simulink model "Test_model_Froce"  (R2024a)
settings: Solver=VariableStepAuto  StartTime=0.0  StopTime=inf  RelTol=1e-3
undefined symbols (not defined in the file or in its folder): X, Y, Z
libraries: sm_lib x62, nesl_utility x21, robotcorelib x4, simulink x1
(part 3 of 3)

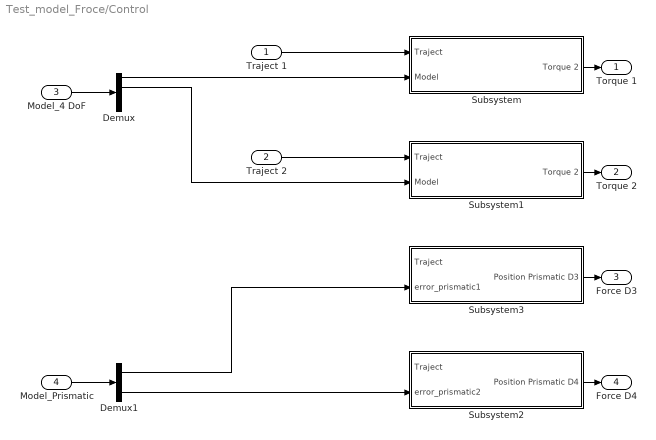
== system Test_model_Froce/Control ==
  Traject 1 : Inport
  Traject 2 : Inport  Port=2
  Model_4 DoF : Inport  Port=3
  Model_Prismatic : Inport  Port=4
  Demux : Demux
  Demux1 : Demux  Outputs=2
  Subsystem : Subsystem
  Subsystem1 : Subsystem
  Subsystem2 : Subsystem
  Subsystem3 : Subsystem
  Torque 1 : Outport
  Torque 2 : Outport  Port=2
  Force D3 : Outport  Port=3
  Force D4 : Outport  Port=4
  wires:
  Subsystem1/1(Torque 2) -> Torque 2/1
  Subsystem/1(Torque 2) -> Torque 1/1
  Subsystem3/1(Position Prismatic D3) -> Force D3/1
  Subsystem2/1(Position Prismatic D4) -> Force D4/1
  Model_4 DoF/1 -> Demux/1
  Demux/1 -> Subsystem/2(Model)
  Demux/2 -> Subsystem1/2(Model)
  Traject 1/1 -> Subsystem/1(Traject)
  Traject 2/1 -> Subsystem1/1(Traject)
  Model_Prismatic/1 -> Demux1/1
  Demux1/1 -> Subsystem3/2(error_prismatic1)
  Demux1/2 -> Subsystem2/2(error_prismatic2)

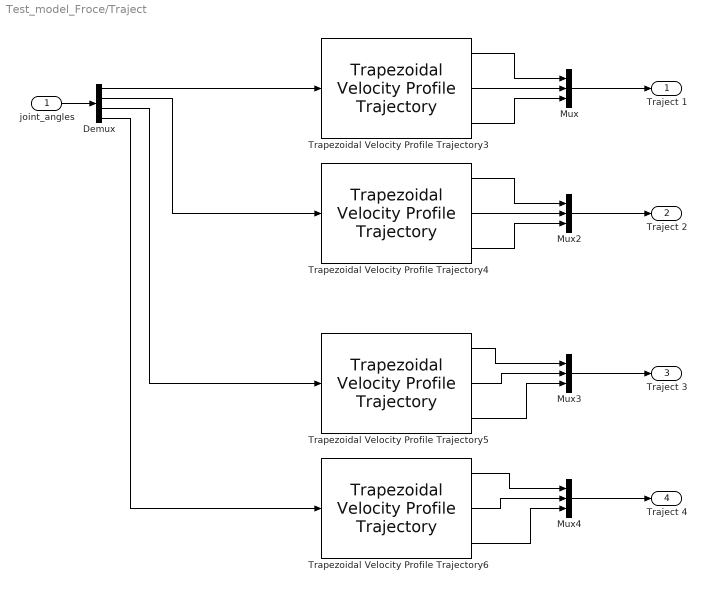
== system Test_model_Froce/Traject ==
  joint_angles : Inport
  Demux : Demux
  Mux{,2..4} (4 alike) : Mux  Inputs=3
  Trapezoidal Velocity Profile Trajectory3 : robotcorelib/Trapezoidal Velocity Profile Trajectory  WaypointSource=Internal  Waypoints=[ 0, 0, 0]  NumParams=0  Parameter1=Peak Velocity  Parameter2=End Time  ParameterSource=Internal  PeakVelocity=[ 2; 2 ]  Acceleration=[ 1; 2 ]  EndTime=[ 1; 1 ]  AccelTime=[ 1; 2 ]  SimulateUsing=Interpreted execution
  Trapezoidal Velocity Profile Trajectory4 : robotcorelib/Trapezoidal Velocity Profile Trajectory  WaypointSource=Internal  Waypoints=[ 0, 0, 0]  NumParams=0  Parameter1=Peak Velocity  Parameter2=End Time  ParameterSource=Internal  PeakVelocity=[ 2; 2 ]  Acceleration=[ 1; 2 ]  EndTime=[ 1; 1 ]  AccelTime=[ 1; 2 ]  SimulateUsing=Interpreted execution
  Trapezoidal Velocity Profile Trajectory5 : robotcorelib/Trapezoidal Velocity Profile Trajectory  WaypointSource=Internal  Waypoints=[ 0, 1, 5]  NumParams=0  Parameter1=Peak Velocity  Parameter2=End Time  ParameterSource=Internal  PeakVelocity=[ 2; 2 ]  Acceleration=[ 1; 2 ]  EndTime=[ 1; 1 ]  AccelTime=[ 1; 2 ]  SimulateUsing=Interpreted execution
  Trapezoidal Velocity Profile Trajectory6 : robotcorelib/Trapezoidal Velocity Profile Trajectory  WaypointSource=Internal  Waypoints=[ 0, 1, 3]  NumParams=0  Parameter1=Peak Velocity  Parameter2=End Time  ParameterSource=Internal  PeakVelocity=[ 2; 2 ]  Acceleration=[ 1; 2 ]  EndTime=[ 1; 1 ]  AccelTime=[ 1; 2 ]  SimulateUsing=Interpreted execution
  Traject 1 : Outport
  Traject 2 : Outport  Port=2
  Traject 3 : Outport  Port=3
  Traject 4 : Outport  Port=4
  wires:
  Trapezoidal Velocity Profile Trajectory5/2 -> Mux3/2
  Trapezoidal Velocity Profile Trajectory3/2 -> Mux/2
  Trapezoidal Velocity Profile Trajectory6/1 -> Mux4/1
  Trapezoidal Velocity Profile Trajectory6/2 -> Mux4/2
  Trapezoidal Velocity Profile Trajectory3/3 -> Mux/3
  Trapezoidal Velocity Profile Trajectory6/3 -> Mux4/3
  Trapezoidal Velocity Profile Trajectory5/3 -> Mux3/3
  Trapezoidal Velocity Profile Trajectory3/1 -> Mux/1
  Trapezoidal Velocity Profile Trajectory4/3 -> Mux2/3
  Trapezoidal Velocity Profile Trajectory4/1 -> Mux2/1
  Trapezoidal Velocity Profile Trajectory4/2 -> Mux2/2
  Trapezoidal Velocity Profile Trajectory5/1 -> Mux3/1
  Mux/1 -> Traject 1/1
  joint_angles/1 -> Demux/1
  Demux/1 -> Trapezoidal Velocity Profile Trajectory3/1
  Demux/2 -> Trapezoidal Velocity Profile Trajectory4/1
  Demux/3 -> Trapezoidal Velocity Profile Trajectory5/1
  Demux/4 -> Trapezoidal Velocity Profile Trajectory6/1
  Mux2/1 -> Traject 2/1
  Mux3/1 -> Traject 3/1
  Mux4/1 -> Traject 4/1

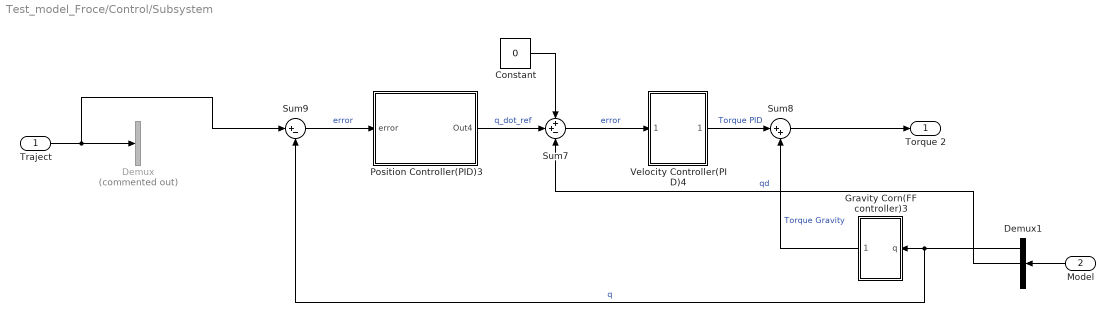
== system Test_model_Froce/Control/Subsystem ==
  Traject : Inport
  Model : Inport  Port=2
  Constant : Constant  Value=0
  Demux : Demux  Commented=on  Outputs=3
  Demux1 : Demux  Outputs=3
  Gravity Corn(FF controller)3 : Subsystem
  Position Controller(PID)3 : Subsystem
  Sum7 : Sum  Inputs=++-
  Sum8 : Sum  Inputs=|++
  Sum9 : Sum  Inputs=|+-
  Velocity Controller(PID)4 : Subsystem
  Torque 2 : Outport
  wires:
  Position Controller(PID)3/1(Out4) -> Sum7/2  "q_dot_ref"
  Gravity Corn(FF controller)3/1(Out1) -> Sum8/2  "Torque Gravity"
  Traject/1 -> Sum9/1, Demux/1
  Velocity Controller(PID)4/1(Out4) -> Sum8/1  "Torque PID"
  Sum7/1 -> Velocity Controller(PID)4/1(error)  "error"
  Sum9/1 -> Position Controller(PID)3/1(error)  "error"
  Sum8/1 -> Torque 2/1
  Model/1 -> Demux1/1
  Demux1/1 -> Sum9/2, Gravity Corn(FF controller)3/1(q)  "q"
  Demux1/2 -> Sum7/3  "qd"
  Constant/1 -> Sum7/1

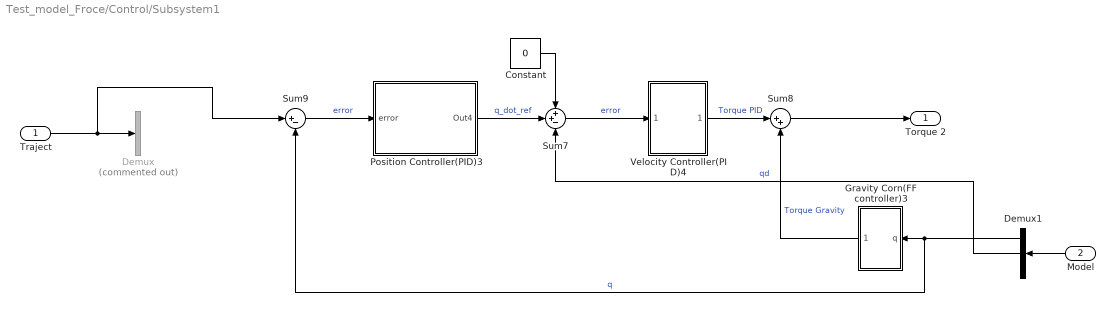
== system Test_model_Froce/Control/Subsystem1 ==
  Traject : Inport
  Model : Inport  Port=2
  Constant : Constant  Value=0
  Demux : Demux  Commented=on  Outputs=3
  Demux1 : Demux  Outputs=3
  Gravity Corn(FF controller)3 : Subsystem
  Position Controller(PID)3 : Subsystem
  Sum7 : Sum  Inputs=++-
  Sum8 : Sum  Inputs=|++
  Sum9 : Sum  Inputs=|+-
  Velocity Controller(PID)4 : Subsystem
  Torque 2 : Outport
  wires:
  Position Controller(PID)3/1(Out4) -> Sum7/2  "q_dot_ref"
  Gravity Corn(FF controller)3/1(Out1) -> Sum8/2  "Torque Gravity"
  Traject/1 -> Sum9/1, Demux/1
  Velocity Controller(PID)4/1(Out4) -> Sum8/1  "Torque PID"
  Sum7/1 -> Velocity Controller(PID)4/1(error)  "error"
  Sum9/1 -> Position Controller(PID)3/1(error)  "error"
  Sum8/1 -> Torque 2/1
  Model/1 -> Demux1/1
  Demux1/1 -> Sum9/2, Gravity Corn(FF controller)3/1(q)  "q"
  Demux1/2 -> Sum7/3  "qd"
  Constant/1 -> Sum7/1

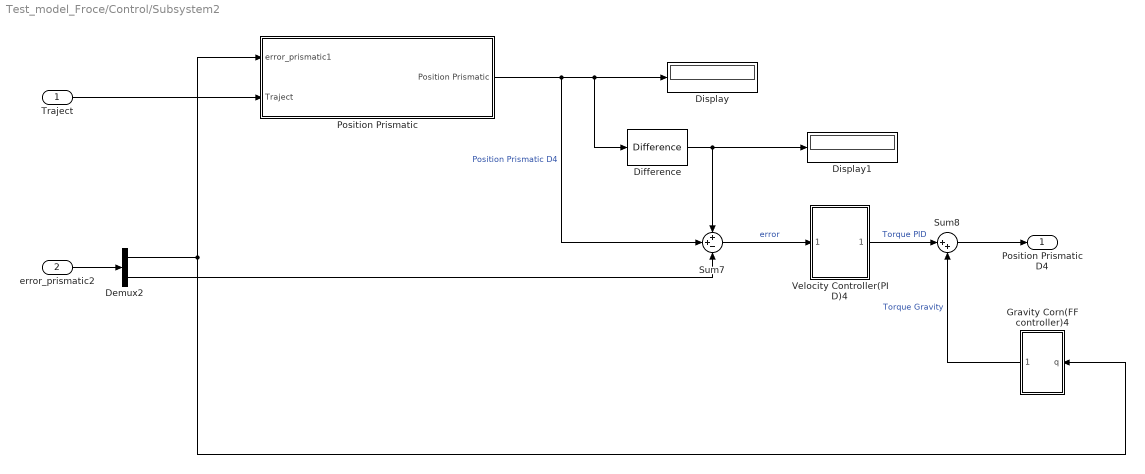
== system Test_model_Froce/Control/Subsystem2 ==
  Traject : Inport
  error_prismatic2 : Inport  Port=2
  Demux2 : Demux  Outputs=2
  Difference : simulink/Discrete/Difference  ICPrevInput=0.0  OutMin=[]  OutMax=[]  OutDataType=fixdt(1, 16)  OutScaling=2^-10  DoSatur=off
  Display : Display
  Display1 : Display
  Gravity Corn(FF controller)4 : Subsystem
  "Position Prismatic " : Subsystem
  Sum7 : Sum  Inputs=++-
  Sum8 : Sum  Inputs=|++
  Velocity Controller(PID)4 : Subsystem
  Position Prismatic D4 : Outport
  wires:
  Gravity Corn(FF controller)4/1(Out1) -> Sum8/2  "Torque Gravity"
  Traject/1 -> "Position Prismatic "/2(Traject)
  Velocity Controller(PID)4/1(Out4) -> Sum8/1  "Torque PID"
  Sum7/1 -> Velocity Controller(PID)4/1(error)  "error"
  "Position Prismatic "/1(Position Prismatic) -> Sum7/2, Difference/1, Display/1  "Position Prismatic D4"
  error_prismatic2/1 -> Demux2/1
  Demux2/1 -> "Position Prismatic "/1(error_prismatic1), Gravity Corn(FF controller)4/1(q)
  Sum8/1 -> Position Prismatic D4/1
  Demux2/2 -> Sum7/3
  Difference/1 -> Sum7/1, Display1/1

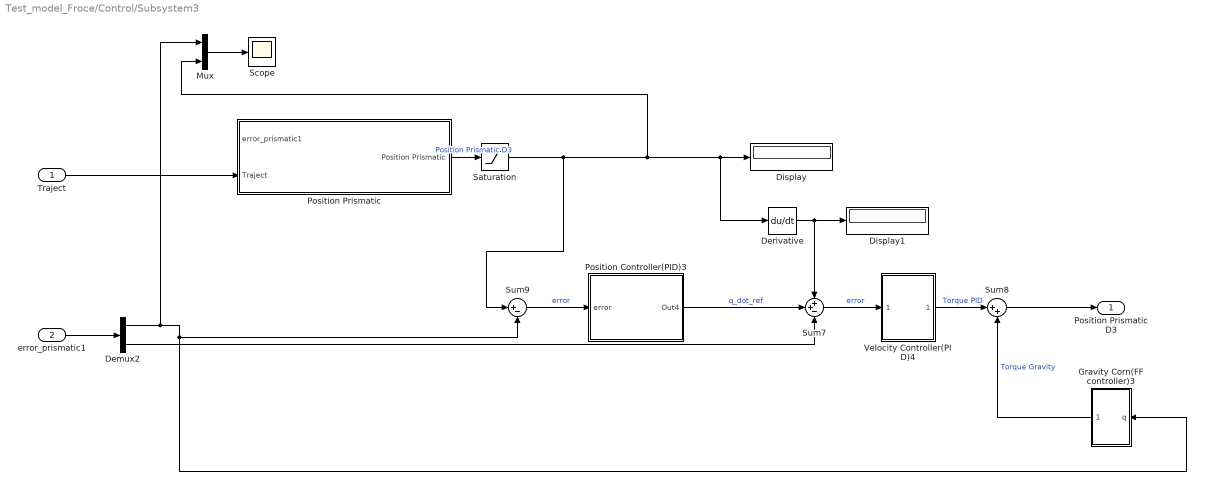
== system Test_model_Froce/Control/Subsystem3 ==
  Traject : Inport
  error_prismatic1 : Inport  Port=2
  Demux2 : Demux  Outputs=2
  Derivative : Derivative
  Display : Display
  Display1 : Display
  Gravity Corn(FF controller)3 : Subsystem
  Mux : Mux  Inputs=2
  Position Controller(PID)3 : Subsystem
  "Position Prismatic " : Subsystem
  Saturation : Saturate  UpperLimit=0.6  LowerLimit=0.25
  Scope : Scope
  Sum7 : Sum  Inputs=++-
  Sum8 : Sum  Inputs=|++
  Sum9 : Sum  Inputs=|+-
  Velocity Controller(PID)4 : Subsystem
  Position Prismatic D3 : Outport
  wires:
  Derivative/1 -> Display1/1, Sum7/1
  Demux2/2 -> Sum7/3
  Sum8/1 -> Position Prismatic D3/1
  Demux2/1 -> Mux/1, Sum9/2, Gravity Corn(FF controller)3/1(q)
  error_prismatic1/1 -> Demux2/1
  "Position Prismatic "/1(Position Prismatic) -> Saturation/1  "Position Prismatic D3"
  Sum7/1 -> Velocity Controller(PID)4/1(error)  "error"
  Velocity Controller(PID)4/1(Out4) -> Sum8/1  "Torque PID"
  Traject/1 -> "Position Prismatic "/2(Traject)
  Gravity Corn(FF controller)3/1(Out1) -> Sum8/2  "Torque Gravity"
  Mux/1 -> Scope/1
  Position Controller(PID)3/1(Out4) -> Sum7/2  "q_dot_ref"
  Sum9/1 -> Position Controller(PID)3/1(error)  "error"
  Saturation/1 -> Sum9/1, Mux/2, Derivative/1, Display/1

== system Test_model_Froce/Control/Subsystem/Gravity Corn(FF controller)3 ==
  note: mgLsin(zeta)
  q : Inport
  Sin : Trigonometry
  mg : Gain  Gain=1*9.80665*1
  Out1 : Outport
  wires:
  Sin/1 -> mg/1
  q/1 -> Sin/1
  mg/1 -> Out1/1

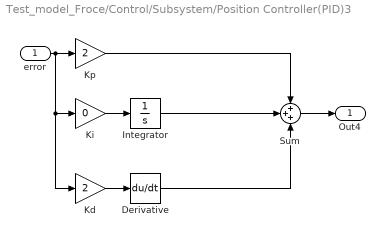
== system Test_model_Froce/Control/Subsystem/Position Controller(PID)3 ==
  error : Inport
  Derivative : Derivative
  Integrator : Integrator
  Kd : Gain  Gain=2
  Ki : Gain  Gain=0
  Kp : Gain  Gain=2
  Sum : Sum  Inputs=+++
  Out4 : Outport
  wires:
  Derivative/1 -> Sum/3
  Ki/1 -> Integrator/1
  Integrator/1 -> Sum/2
  Kd/1 -> Derivative/1
  Kp/1 -> Sum/1
  error/1 -> Kd/1, Ki/1, Kp/1
  Sum/1 -> Out4/1

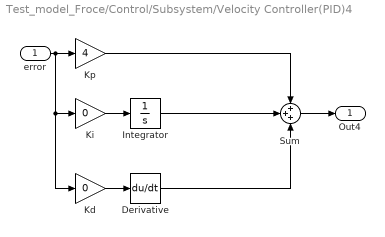
== system Test_model_Froce/Control/Subsystem/Velocity Controller(PID)4 ==
  error : Inport
  Derivative : Derivative
  Integrator : Integrator
  Kd : Gain  Gain=0
  Ki : Gain  Gain=0
  Kp : Gain  Gain=4
  Sum : Sum  Inputs=+++
  Out4 : Outport
  wires:
  Derivative/1 -> Sum/3
  Ki/1 -> Integrator/1
  Integrator/1 -> Sum/2
  Kd/1 -> Derivative/1
  Kp/1 -> Sum/1
  error/1 -> Kd/1, Ki/1, Kp/1
  Sum/1 -> Out4/1

== system Test_model_Froce/Control/Subsystem1/Gravity Corn(FF controller)3 ==
  note: mgLsin(zeta)
  q : Inport
  Sin : Trigonometry
  mg : Gain  Gain=1*9.80665*1
  Out1 : Outport
  wires:
  Sin/1 -> mg/1
  q/1 -> Sin/1
  mg/1 -> Out1/1

== system Test_model_Froce/Control/Subsystem1/Position Controller(PID)3 ==
  error : Inport
  Derivative : Derivative
  Integrator : Integrator
  Kd : Gain  Gain=2
  Ki : Gain  Gain=0
  Kp : Gain  Gain=2
  Sum : Sum  Inputs=+++
  Out4 : Outport
  wires:
  Derivative/1 -> Sum/3
  Ki/1 -> Integrator/1
  Integrator/1 -> Sum/2
  Kd/1 -> Derivative/1
  Kp/1 -> Sum/1
  error/1 -> Kd/1, Ki/1, Kp/1
  Sum/1 -> Out4/1

== system Test_model_Froce/Control/Subsystem1/Velocity Controller(PID)4 ==
  error : Inport
  Derivative : Derivative
  Integrator : Integrator
  Kd : Gain  Gain=0
  Ki : Gain  Gain=0
  Kp : Gain  Gain=4
  Sum : Sum  Inputs=+++
  Out4 : Outport
  wires:
  Derivative/1 -> Sum/3
  Ki/1 -> Integrator/1
  Integrator/1 -> Sum/2
  Kd/1 -> Derivative/1
  Kp/1 -> Sum/1
  error/1 -> Kd/1, Ki/1, Kp/1
  Sum/1 -> Out4/1

== system Test_model_Froce/Control/Subsystem2/Gravity Corn(FF controller)4 ==
  note: mgLsin(zeta)
  q : Inport
  Sin : Trigonometry
  mg : Gain  Gain=1*9.80665*1
  Out1 : Outport
  wires:
  Sin/1 -> mg/1
  q/1 -> Sin/1
  mg/1 -> Out1/1

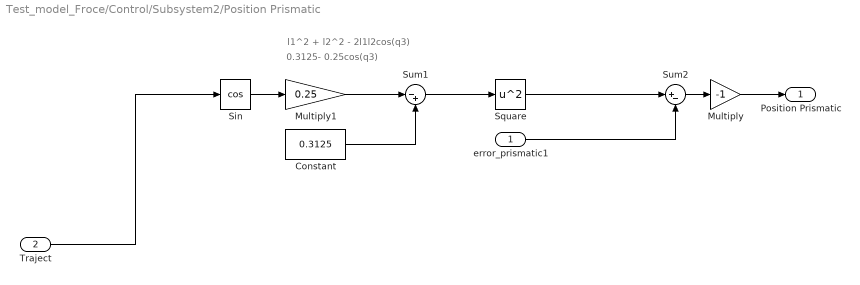
== system Test_model_Froce/Control/Subsystem2/Position Prismatic  ==
  note: l1^2 + l2^2 - 2l1l2cos(q3)
  note: 0.3125- 0.25cos(q3)
  error_prismatic1 : Inport
  Traject : Inport  Port=2
  Constant : Constant  Value=0.3125
  Multiply : Gain  Gain=-1
  Multiply1 : Gain  Gain=0.25
  Sin : Trigonometry  Operator=cos
  Square : Math  Operator=square
  Sum1 : Sum  Inputs=|-+
  Sum2 : Sum  Inputs=|+-
  Position Prismatic : Outport
  wires:
  Sum1/1 -> Square/1
  Square/1 -> Sum2/1
  Constant/1 -> Sum1/2
  Sin/1 -> Multiply1/1
  error_prismatic1/1 -> Sum2/2
  Sum2/1 -> Multiply/1
  Traject/1 -> Sin/1
  Multiply1/1 -> Sum1/1
  Multiply/1 -> Position Prismatic/1

== system Test_model_Froce/Control/Subsystem2/Velocity Controller(PID)4 ==
  error : Inport
  Derivative : Derivative
  Integrator : Integrator
  Kd : Gain  Gain=0
  Ki : Gain  Gain=0
  Kp : Gain  Gain=20
  Sum : Sum  Inputs=+++
  Out4 : Outport
  wires:
  Derivative/1 -> Sum/3
  Ki/1 -> Integrator/1
  Integrator/1 -> Sum/2
  Kd/1 -> Derivative/1
  Kp/1 -> Sum/1
  error/1 -> Kd/1, Ki/1, Kp/1
  Sum/1 -> Out4/1

== system Test_model_Froce/Control/Subsystem3/Gravity Corn(FF controller)3 ==
  note: mgLsin(zeta)
  q : Inport
  Sin : Trigonometry
  mg : Gain  Gain=1*9.80665*1
  Out1 : Outport
  wires:
  mg/1 -> Out1/1
  q/1 -> Sin/1
  Sin/1 -> mg/1

== system Test_model_Froce/Control/Subsystem3/Position Controller(PID)3 ==
  error : Inport
  Derivative : Derivative
  Integrator : Integrator
  Kd : Gain  Gain=2
  Ki : Gain  Gain=0
  Kp : Gain  Gain=10
  Sum : Sum  Inputs=+++
  Out4 : Outport
  wires:
  Derivative/1 -> Sum/3
  Ki/1 -> Integrator/1
  Integrator/1 -> Sum/2
  Kd/1 -> Derivative/1
  Kp/1 -> Sum/1
  error/1 -> Kd/1, Ki/1, Kp/1
  Sum/1 -> Out4/1

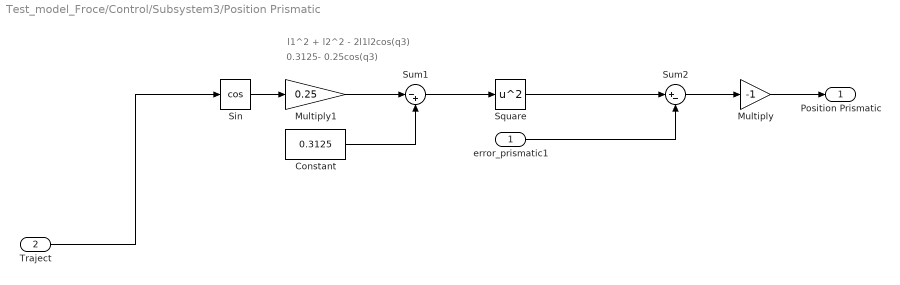
== system Test_model_Froce/Control/Subsystem3/Position Prismatic  ==
  note: 0.3125- 0.25cos(q3)
  note: l1^2 + l2^2 - 2l1l2cos(q3)
  error_prismatic1 : Inport
  Traject : Inport  Port=2
  Constant : Constant  Value=0.3125
  Multiply : Gain  Gain=-1
  Multiply1 : Gain  Gain=0.25
  Sin : Trigonometry  Operator=cos
  Square : Math  Operator=square
  Sum1 : Sum  Inputs=|-+
  Sum2 : Sum  Inputs=|+-
  Position Prismatic : Outport
  wires:
  Multiply1/1 -> Sum1/1
  Traject/1 -> Sin/1
  Sum2/1 -> Multiply/1
  Sin/1 -> Multiply1/1
  Constant/1 -> Sum1/2
  Square/1 -> Sum2/1
  Sum1/1 -> Square/1
  error_prismatic1/1 -> Sum2/2
  Multiply/1 -> Position Prismatic/1

== system Test_model_Froce/Control/Subsystem3/Velocity Controller(PID)4 ==
  error : Inport
  Derivative : Derivative
  Integrator : Integrator
  Kd : Gain  Gain=0
  Ki : Gain  Gain=0
  Kp : Gain  Gain=4
  Sum : Sum  Inputs=+++
  Out4 : Outport
  wires:
  Sum/1 -> Out4/1
  error/1 -> Kp/1, Ki/1, Kd/1
  Kp/1 -> Sum/1
  Kd/1 -> Derivative/1
  Integrator/1 -> Sum/2
  Ki/1 -> Integrator/1
  Derivative/1 -> Sum/3

== matlab function Test_model_Froce/MATLAB Function1 ==
  data: joint_angles input; x output; y output; z output; phi output
function [x, y, z, phi] = FK_Simulink(joint_angles)
    % FK_Simulink: Calculates the position and orientation of the end effector for a 4-DOF manipulator

    % Lengths of the links
    L1 = 0.25; % Link 1
    L2 = 1; % Link 2
    L3 = 1.5; % Link 3
    L4 = 0.75; % Link 4 (End Effector)

    % Extract joint angles
    q1 = joint_angles(1); % Joint 1 (base rotation)
    q2 = joint_angles(2); % Joint 2 (shoulder rotation)
    q3 = joint_angles(3); % Joint 3 (elbow rotation)
    q4 = joint_angles(4); % Joint 4 (end effector orientation)

    % Transformation Matrices
    % Transform from base frame to end effector
    % Transformation for Joint 1 (Rotation around the base)
    T1 = [cos(q1), -sin(q1), 0, -0.2;
          sin(q1),  cos(q1), 0,    0;
                0,        0, 1,   L1;
                0,        0, 0,   1];
     %T1 = [1, 0, 0, -0.2;
          %0, 1, 0, 0;
          %0, 0, 1, L1;
          %0, 0, 0, 1];

    % Transformation for Joint 2 (shoulder)
    T2 = [cos(q2), -sin(q2), 0, 0;
                0,        0, 1, 0;
          sin(q2),  cos(q2), 0, 0;
                0,        0, 0, 1];
     %T2 = [0, -1, 0, 0;
           %0, 0, 1, 0;
          %1, 0, 0, 0;
          %0, 0, 0, 1];

    % Transformation for Joint 3 (elbow)
    T3 = [cos(q3), -sin(q3), 0, L2;
          sin(q3),  cos(q3), 0,  0;
                0,        0, 1,  0;
                0,        0, 0, 1];
     %T3 = [1, 0, 0, L2;
          %0, 1, 0, 0;
          %0, 0, 1, 0;
          %0, 0, 0, 1];

    % Transformation for Joint 4 (end effector orientation)
    T4 = [cos(q4), -sin(q4), 0, L3;
          sin(q4),  cos(q4), 0,  0;
                0,        0, 1,  0;
                0,        0, 0, 1];
     %T4 = [1, 0, 0, L3;
          %0, 1, 0, 0;
          %0, 0, 1, 0;
          %0, 0, 0, 1];

    T5 = [1, 0, 0, L4;
          0, 1, 0, 0;
          0, 0, 1, 0;
          0, 0, 0, 1];
    %T5 = [1, 0, 0, L4;
          %0, 1, 0, 0;
          %0, 0, 1, 0;
          %0, 0, 0, 1];

    % Final transformation from the base to end effector
    T = T1 * T2 * T3 * T4 * T5;

    % Extract position from the final transformation matrix
    x = T(1, 4); % x-position of the end effector
    y = T(2, 4); % y-position of the end effector
    z = T(3, 4); % z-position of the end effector

    % Extract orientation (phi) from the transformation matrix
    phi = atan2(T(2, 1), T(1, 1)); % Rotation around the z-axis (orientation of the end effector)
end

== matlab function Test_model_Froce/MATLAB Function ==
  data: x_target input; theta output; y_target input; z_target input; L1 input; L2 input; L3 input; L4 input
function theta = inverse_kinematics(x_target, y_target, z_target, L1, L2, L3, L4)
% Inverse Kinematics for a 4-DOF Robot Arm
% Inputs:
% x_target, y_target, z_target: Target position in 3D space
% L1, L2, L3, L4: Lengths of the robot arm links
%
% Output:
% theta: Joint angles [theta1, theta2, theta3, theta4]

    % Initialize joint angles
    theta = zeros(4, 1);
    
    % Solve for theta1 (rotation in base plane)
    theta(1) = atan2(y_target, x_target);

    % Calculate r (distance in the horizontal plane)
    r = sqrt(x_target^2 + y_target^2);
    
    % Solve for theta2 and theta3 using geometry
    z_eff = z_target - L1; % Effective height
    d = sqrt(r^2 + z_eff^2); % Distance to target from base joint
    
    % Check if the target is reachable
    if d > (L2 + L3)
        error('Target is out of reach');
    end

    % Use law of cosines to solve for theta2 and theta3
    cos_theta2 = (L2^2 + d^2 - L3^2) / (2 * L2 * d);
    sin_theta2 = sqrt(1 - cos_theta2^2); % Assuming positive solution
    theta(2) = atan2(z_eff, r) + atan2(sin_theta2, cos_theta2);

    cos_theta3 = (L2^2 + L3^2 - d^2) / (2 * L2 * L3);
    sin_theta3 = sqrt(1 - cos_theta3^2); % Assuming positive solution
    theta(3) = atan2(sin_theta3, cos_theta3);

    % Solve for theta4 (orientation of the end effector)
    theta(4) = 0; % Assuming no additional orientation control for simplicity
end

== matlab function Test_model_Froce/MATLAB Function2 ==
  data: q input; T output; L1 input; L2 input; L3 input; L4 input
function T = forward_kinematics(q, L1, L2, L3, L4)
    coder.extrinsic('rtb.DHRobot', 'rtb.RevoluteMDH', 'spatialmath.SE3');
    
    % สร้างโมเดลหุ่นยนต์
    robot = rtb.DHRobot([
        rtb.RevoluteMDH(0, 0, L1, 0),
        rtb.RevoluteMDH(0, pi/2, 0, 0),
        rtb.RevoluteMDH(-L2, 0, 0, 0),
        rtb.RevoluteMDH(-L3, 0, 0, 0),
        rtb.RevoluteMDH(-L4, 0, 0, 0)
    ], 'name', 'Test');
    
    % คำนวณ FK
    T = robot.fkine(q);
    T = double(T.t); % แปลงให้เหลือแค่ Translation
end

== matlab function Test_model_Froce/MATLAB Function3 ==
  data: target input; q output; L1 input; L2 input; L3 input; L4 input
function q = inverse_kinematics(target, L1, L2, L3, L4)
    coder.extrinsic('rtb.DHRobot', 'rtb.RevoluteMDH', 'spatialmath.SE3');
    
    % สร้างโมเดลหุ่นยนต์
    robot = rtb.DHRobot([
        rtb.RevoluteMDH(0, 0, L1, 0),
        rtb.RevoluteMDH(0, pi/2, 0, 0),
        rtb.RevoluteMDH(-L2, 0, 0, 0),
        rtb.RevoluteMDH(-L3, 0, 0, 0),
        rtb.RevoluteMDH(-L4, 0, 0, 0)
    ], 'name', 'HW_2');
    
    % สร้างเป้าหมาย
    T = SE3(target);
    
    % คำนวณ IK
    sol = robot.ikine(T);
    q = sol.q; % ผลลัพธ์มุมข้อต่อ
end
